simulink model "pid_10"  (R2022a)
settings: Solver=FixedStepAuto  StartTime=0.0  StopTime=12.0  FixedStep=0.1  RelTol=1e-3  EnableMultiTasking=on
libraries: mbedblockslib x27, simulink x3, hdlsllib x2, slctrlblks x1, slpidlib x1
(part 1 of 2)
settings Model: PacingRate=0.750000  ExtModeTrigDuration=10  Creator=MATLAB  LastModifiedBy=FUGAZI
settings SolverCC: AutoInsertRateTranBlk=on
settings OptimizationCC: EnhancedBackFolding=on  PassReuseOutputArgsAs=Individual arguments  ZeroExternalMemoryAtStartup=off  ZeroInternalMemoryAtStartup=off  MaxStackSize=64  OptimizeBlockOrder=speed  DifferentSizesBufferReuse=on  OptimizationCustomize=off  EfficientTunableParamExpr=on
settings DebuggingCC: ParameterTunabilityLossMsg=error
settings HardwareCC: ProdBitPerPointer=32  ProdBitPerSizeT=32  ProdBitPerPtrDiffT=32  ProdLargestAtomicInteger=Long  ProdLargestAtomicFloat=Double  ProdWordSize=32  ProdLongLongMode=on  ProdHWDeviceType=ARM Compatible->ARM Cortex
settings SFSimCC: MATLABDynamicMemAlloc=off
settings RTWCC: SystemTargetFile=ert.tlc  HardwareBoard=STM32 Nucleo L476RG  TemplateMakefile=ert_default_tmf  Toolchain=GNU Tools for ARM Embedded Processors
settings CodeAppCC: ForceParamTrailComments=on  IgnoreCustomStorageClasses=off  OperatorAnnotations=on  SimulinkDataObjDesc=on  SFDataObjDesc=on  InsertBlockDesc=on
settings ERTTargetCC: SupportContinuousTime=on  ExtModeTransport=3  ExtModeStaticAlloc=on  ExtModeStaticAllocSize=2000  ExtModeMexFile=ext_xcp  ExtModeIntrfLevel=Level2 - Open

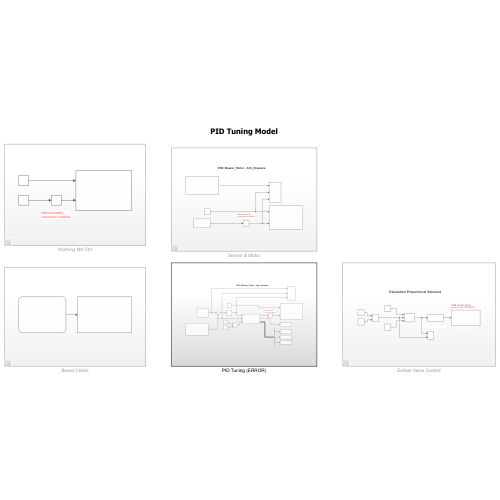
[thumbnail: Simulink's stored preview of the top-level diagram]
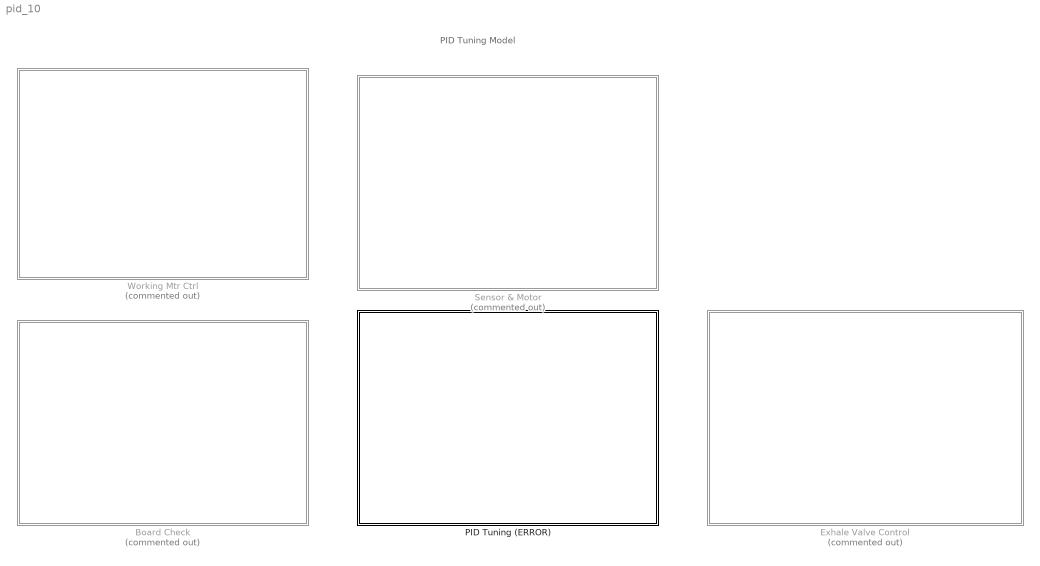
== system pid_10 ==
  note: PID Tuning Model
  Board Check : Subsystem  Commented=on
  Exhale Valve Control : Subsystem  Commented=on
  PID Tuning (ERROR) : Subsystem
  Sensor & Motor : Subsystem  Commented=on
  Working Mtr Ctrl : Subsystem  Commented=on

== system pid_10/Board Check ==
  Start-Up : Stateflow chart  TreatAsAtomicUnit=on
  SubSystem Relays : Subsystem
  wires:
  Start-Up/1(LED) -> SubSystem Relays/1(LED)

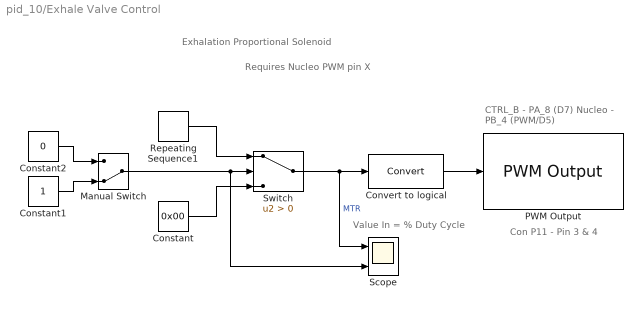
== system pid_10/Exhale Valve Control ==
  note: Exhalation Proportional Solenoid
  note: Value In = % Duty Cycle
  note: Con P11 - Pin 3 & 4
  note: Requires Nucleo PWM pin X
  note: CTRL_B - PA_8 (D7)
      | Nucleo - PB_4 (PWM/D5)
  Constant : Constant  Value=0x00
  Constant1 : Constant
  Constant2 : Constant  Value=0
  Convert to logical : DataTypeConversion  SaturateOnIntegerOverflow=off  RndMeth=Floor
  Manual Switch : ManualSwitch  CurrentSetting=0
  PWM Output : mbedblockslib/PWM Output  Pin=PB_4  EnableInputFrequency=off  InitialFrequency=500  InitialDutyCycle=85  NotificationType=None
      settings: SourceProductBaseCode=MICROBIT,NUCLEO,STMICRODIS
  Repeating Sequence1 : simulink/Sources/Repeating Sequence  rep_seq_t=[0 1.3 1.4 2.5 2.6]  rep_seq_y=[15 15 71 71 15]
  Scope : Scope  NumInputPorts=2
  Switch : Switch  Criteria=u2 > Threshold  SaturateOnIntegerOverflow=off  InputSameDT=off
  wires:
  Manual Switch/1 -> Scope/2, Switch/2
  Convert to logical/1 -> PWM Output/1
  Switch/1 -> Scope/1, Convert to logical/1  "MTR"
  Repeating Sequence1/1 -> Switch/1
  Constant/1 -> Switch/3
  Constant1/1 -> Manual Switch/2
  Constant2/1 -> Manual Switch/1

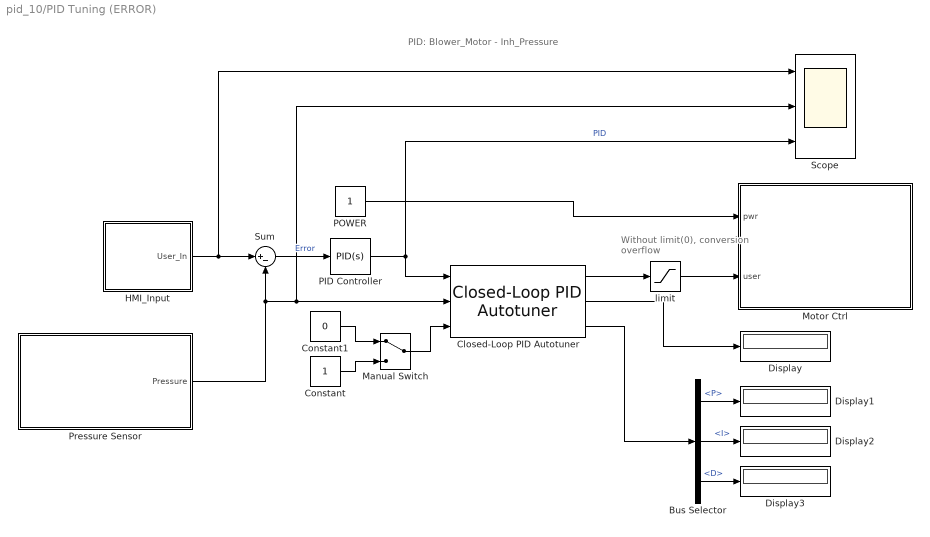
== system pid_10/PID Tuning (ERROR) ==
  note: Without limit(0),
      | conversion overflow
  note: PID: Blower_Motor - Inh_Pressure
  Bus Selector : BusSelector  OutputSignals=P,I,D
  Closed-Loop PID Autotuner : slctrlblks/Closed-Loop PID Autotuner  PIDType=PI  PIDForm=Parallel  TimeDomain=discrete-time  DiscreteTs=0.1  TuningTs=0.2  UseTuningTs=off  IntegratorFormula=Forward Euler  FilterFormula=Forward Euler  ContinuousTs=0.02  Bandwidth=1  UseExternalWC=off  TargetPM=60  UseExternalPM=off  UseExternalAchievedPM=off  ExperimentMode=Superposition  PlantType=Stable  PlantSign=Positive  AmpSine=1  UseExternalAmpSine=off  UseExternalFRD=off  UseExternalU0=off  UseCompanion=off  NotDeployTuningModule=off  UsePLCCoder=off  OutputMode=control action + perturbation  BlockDataType=double  UseConnectedPID=on  blockpath=[]  tunedP=0  tunedI=0  tunedD=0  tunedN=100  tunedPM=0  EstimationWindowSize=3  UseExternalTuningParams=off  OutputChoice=VariantCandD  SingleMultiRateVariant=SingleSamplingRate  ExperimentModeVariant=VariantSuperimposed  NumEstimationPeriods=4  NumSettlingPeriods=2
      settings: SourceProductBaseCode=SD
  Constant : Constant
  Constant1 : Constant  Value=0
  Display{,1..3} (4 alike) : Display
  HMI_Input : Subsystem
  Manual Switch : ManualSwitch
  Motor Ctrl : Subsystem
  PID Controller : slpidlib/PID Controller  Controller=PID  Form=Parallel  TimeDomain=Continuous-time  UseExternalTs=off  SampleTime=-1  IntegratorMethod=Forward Euler  FilterMethod=Forward Euler  ControllerParametersSource=internal  P=2  I=2  UseKiTs=off  D=1.5  N=280  UseFilter=on  TunerSelectOption=Transfer Function Based (PID Tuner App)  InitialConditionSource=internal  InitialConditionForIntegrator=0  InitialConditionForFilter=0  DifferentiatorICPrevScaledInput=0  ExternalReset=none  TrackingMode=off  Kt=1  LimitOutput=off  SatLimitsSource=internal  UpperSaturationLimit=inf  LowerSaturationLimit=-inf  LinearizeAsGain=on  AntiWindupMode=none  Kb=1  POutMin=[]  POutMax=[]  IOutMin=[]  IOutMax=[]  DOutMin=[]  DOutMax=[]  NOutMin=[]  NOutMax=[]  SumOutMin=[]  SumOutMax=[]  SaturationOutMin=[]  SaturationOutMax=[]  PParamMin=[]  PParamMax=[]  IParamMin=[]  IParamMax=[]  DParamMin=[]  DParamMax=[]  NParamMin=[]  NParamMax=[]  KbParamMin=[]  KbParamMax=[]  KtParamMin=[]  KtParamMax=[]  KbOutMin=[]  KbOutMax=[]  KtOutMin=[]  KtOutMax=[]  IntegratorOutMin=[]  IntegratorOutMax=[]  FilterOutMin=[]  FilterOutMax=[]  SumI1OutMin=[]  SumI1OutMax=[]  SumI2OutMin=[]  SumI2OutMax=[]  SumI3OutMin=[]  SumI3OutMax=[]  SumI4OutMin=[]  SumI4OutMax=[]  SumDOutMin=[]  SumDOutMax=[]  DifferentiatorOutMin=[]  DifferentiatorOutMax=[]  FilterDiffOutCoefMin=[]  FilterDiffOutCoefMax=[]  ReciprocalOutMin=[]  ReciprocalOutMax=[]  SumDenOutMin=[]  SumDenOutMax=[]  SumNumOutMin=[]  SumNumOutMax=[]  DivideOutMin=[]  DivideOutMax=[]  UdiffTsProdOutMin=[]  UdiffTsProdOutMax=[]  NTsProdOutMin=[]  NTsProdOutMax=[]  UintegralTsProdOutMin=[]  UintegralTsProdOutMax=[]  UngainTsProdOutMin=[]  UngainTsProdOutMax=[]  IntegratorContinuousStateAttributes=''  IntegratorStateMustResolveToSignalObject=off  IntegratorRTWStateStorageClass=Auto  FilterContinuousStateAttributes=''  FilterStateMustResolveToSignalObject=off  FilterRTWStateStorageClass=Auto  ParallelPVariant=InternalParameters  IdealPVariant=Disabled  IVariant=InternalParameters  DVariant=InternalParameters  IntegratorVariant=Continuous  SatVariant=Disabled  AWVariant=Passthrough  PCopyVariant=Disabled  TRVariant=Disabled  FdbkBlocksVariant=Forward  IdealPFdbkVariant=Disabled  SatFdbkVariant=Disabled  DerivativeFilterVariant=ContFilter  NVariant=InternalParameters  NCopyVariant=Disabled  FilterICVariant=InternalICsFilter  IntegratorICVariant=InternalICs  ExternalResetVariant=Disabled  TRSumVariant=Passthrough  SumFdbkVariant=Disabled  SumVariant=Sum_PID  TsampFilterVariant=InternalTs  TsampNgainVariant=Passthrough  TsampIntegralVariant=Passthrough  ExternalSaturationOutDataTypeStr=Inherit: Same as second input  aMode=0
  POWER : Constant
  Pressure Sensor : Subsystem
  Scope : Scope  NumInputPorts=3
  Sum : Sum  Inputs=|+-
  limit : Saturate  UpperLimit=254  LowerLimit=0
  wires:
  POWER/1 -> Motor Ctrl/1(pwr)
  Bus Selector/3 -> Display3/1  "<D>"
  Pressure Sensor/1(Pressure) -> Sum/2, Scope/2, Closed-Loop PID Autotuner/2
  Closed-Loop PID Autotuner/2 -> Display/1
  Closed-Loop PID Autotuner/1 -> limit/1
  Constant1/1 -> Manual Switch/1
  Bus Selector/2 -> Display2/1  "<I>"
  Bus Selector/1 -> Display1/1  "<P>"
  HMI_Input/1(User_In) -> Scope/1, Sum/1
  Closed-Loop PID Autotuner/3 -> Bus Selector/1
  Manual Switch/1 -> Closed-Loop PID Autotuner/3
  PID Controller/1 -> Closed-Loop PID Autotuner/1, Scope/3  "PID"
  Constant/1 -> Manual Switch/2
  Sum/1 -> PID Controller/1  "Error"
  limit/1 -> Motor Ctrl/2(user)

== system pid_10/Sensor & Motor ==
  note: PID: Blower_Motor - Inh_Pressure
  note: Without limit(0),
      | conversion overflow
  HMI_Input : Subsystem
  Motor Ctrl : Subsystem
  POWER : Constant
  Pressure Sensor : Subsystem
  Scope : Scope  NumInputPorts=3
  limit : Saturate  UpperLimit=254  LowerLimit=0
  wires:
  limit/1 -> Scope/3, Motor Ctrl/2(user)
  POWER/1 -> Scope/2, Motor Ctrl/1(pwr)
  HMI_Input/1(User_In) -> limit/1
  Pressure Sensor/1(Pressure) -> Scope/1

== system pid_10/Working Mtr Ctrl ==
  note: Without limit(0),
      | conversion overflow
  Constant : Constant
  Constant1 : Constant  Value=120
  Motor Ctrl : Subsystem
  limit : Saturate  UpperLimit=254  LowerLimit=0
  wires:
  limit/1 -> Motor Ctrl/2(user)
  Constant1/1 -> limit/1
  Constant/1 -> Motor Ctrl/1(pwr)

== system pid_10/Board Check/SubSystem Relays ==
  note: Logic Switching Sub-Systems
  note: Simulation Port
  note: Status LED PB_0
      | Nucleo PA_5
  LED : Inport
  Data Type Conversion1 : DataTypeConversion  SaturateOnIntegerOverflow=off  RndMeth=Floor
  Digital Write2 : mbedblockslib/Digital Write  Pin=PA_5  Direction=output
      settings: SourceProductBaseCode=MICROBIT,NUCLEO,STMICRODIS
  Scope : Scope
  wires:
  LED/1 -> Data Type Conversion1/1
  Data Type Conversion1/1 -> Digital Write2/1, Scope/1

== system pid_10/PID Tuning (ERROR)/HMI_Input ==
  Constant : Constant  Value=8
  Continuous Input : DiscretePulseGenerator  Commented=on  PulseType=Time based  Amplitude=61  Period=10  PulseWidth=50
  Step Input : Step  Before=6  After=21  SampleTime=5
  Varying Inputs : simulink/Sources/Repeating Sequence Stair  Commented=on  OutValues=[1638 8191 16383 8191 1638].'  tsamp=2  OutMin=[]  OutMax=[]  OutDataTypeStr=double  OutputDataTypeScalingMode=double  OutDataType=fixdt(0,8)  ConRadixGroup=Best Precision: Vector-wise  OutScaling=2^-12
  User_In : Outport
  wires:
  Constant/1 -> User_In/1

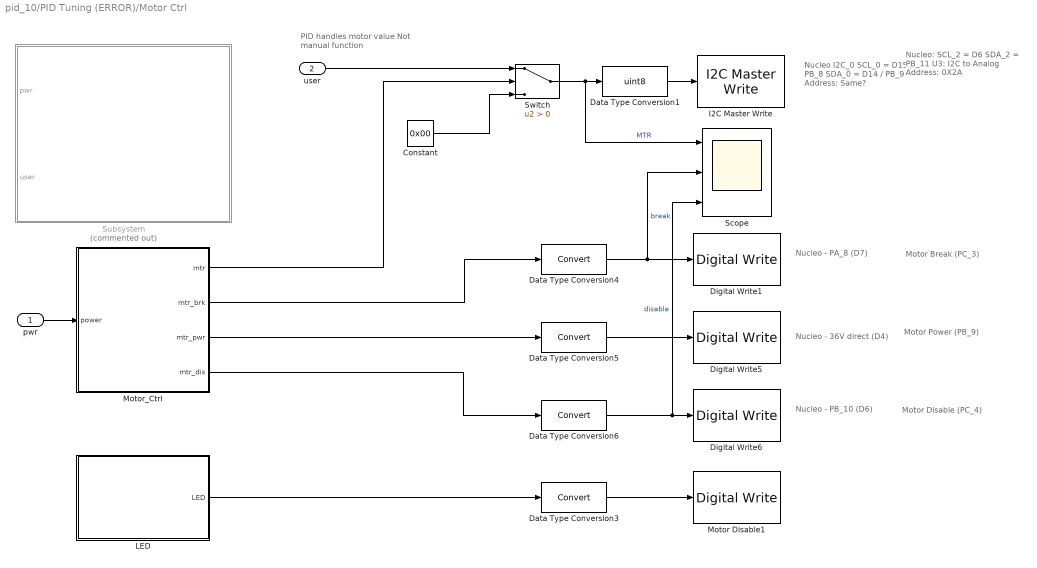
== system pid_10/PID Tuning (ERROR)/Motor Ctrl ==
  note: Nucleo I2C_0
      | SCL_0 = D15 / PB_8
      | SDA_0 = D14 / PB_9
      | Address: Same?
  note: PID handles motor value
      | Not manual function
  note: Motor Power
      | (PB_9)
  note: Motor Break
      | (PC_3)
  note: Nucleo:
      | SCL_2 = D6
      | SDA_2 = PB_11
      | U3: I2C to Analog
      | Address: 0X2A
  note: Nucleo - 36V direct
      | (D4)
  note: Motor Disable
      | (PC_4)
  note: Nucleo - PA_8
      | (D7)
  note: Nucleo - PB_10
      | (D6)
  pwr : Inport
  user : Inport  Port=2
  Constant : Constant  Value=0x00
  Data Type Conversion1 : DataTypeConversion  OutDataTypeStr=uint8  SaturateOnIntegerOverflow=off  RndMeth=Floor
  Data Type Conversion{3..6} (4 alike) : DataTypeConversion  SaturateOnIntegerOverflow=off  RndMeth=Floor
  Digital Write1 : mbedblockslib/Digital Write  Pin=PA_8  Direction=output
      settings: SourceProductBaseCode=MICROBIT,NUCLEO,STMICRODIS
  Digital Write5 : mbedblockslib/Digital Write  Pin=PB_5  Direction=output
      settings: SourceProductBaseCode=MICROBIT,NUCLEO,STMICRODIS
  Digital Write6 : mbedblockslib/Digital Write  Pin=PB_10  Direction=output
      settings: SourceProductBaseCode=MICROBIT,NUCLEO,STMICRODIS
  I2C Master Write : mbedblockslib/I2C Master Write  I2CModule=0  Mode=Master  SlaveAddress=uint8(hex2dec('2A'))  SlaveByteOrder=BigEndian  Direction=Transmitter  RegisterAddressMode=on  RegisterAddress=uint8(hex2dec('10'))  SlaveDataType=uint8  DataLength=2  NoAck=off  RepeatedStart=off  OutputStatus=off
      settings: SourceProductBaseCode=MICROBIT,NUCLEO,STMICRODIS
  LED : Stateflow chart  TreatAsAtomicUnit=on
  Motor Disable1 : mbedblockslib/Digital Write  Pin=PA_5  Direction=output
      settings: SourceProductBaseCode=MICROBIT,NUCLEO,STMICRODIS
  Motor_Ctrl : Stateflow chart  TreatAsAtomicUnit=on
  Scope : Scope  NumInputPorts=3
  Subsystem : Subsystem  Commented=on
  Switch : Switch  Criteria=u2 > Threshold  SaturateOnIntegerOverflow=off  InputSameDT=off
  wires:
  Motor_Ctrl/3(mtr_pwr) -> Data Type Conversion5/1
  Constant/1 -> Switch/3
  Data Type Conversion3/1 -> Motor Disable1/1
  LED/1(LED) -> Data Type Conversion3/1
  Switch/1 -> Scope/1, Data Type Conversion1/1  "MTR"
  user/1 -> Switch/1
  Data Type Conversion5/1 -> Digital Write5/1
  Data Type Conversion4/1 -> Scope/2, Digital Write1/1  "break"
  pwr/1 -> Motor_Ctrl/1(power)
  Motor_Ctrl/1(mtr) -> Switch/2
  Data Type Conversion6/1 -> Scope/3, Digital Write6/1  "disable"
  Motor_Ctrl/4(mtr_dis) -> Data Type Conversion6/1
  Data Type Conversion1/1 -> I2C Master Write/1
  Motor_Ctrl/2(mtr_brk) -> Data Type Conversion4/1

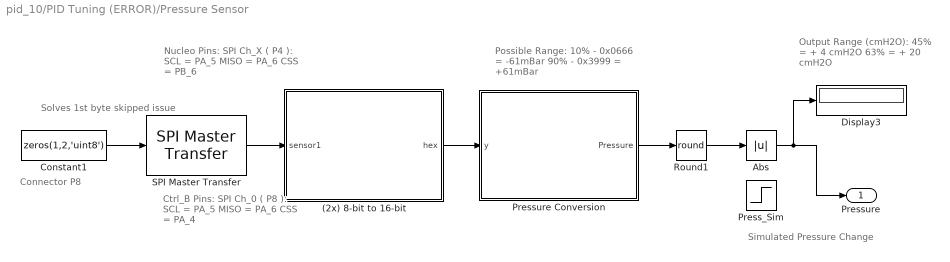
== system pid_10/PID Tuning (ERROR)/Pressure Sensor ==
  note: Ctrl_B Pins:
      | SPI Ch_0 ( P8 ):
      | SCL = PA_5
      | MISO = PA_6
      | CSS = PA_4
  note: Possible Range:
      | 10% - 0x0666 = -61mBar
      | 90% - 0x3999 = +61mBar
  note: Connector P8
  note: Solves 1st byte
      | skipped issue
  note: Output Range (cmH2O):
      | 45% = + 4 cmH2O
      | 63% = + 20 cmH2O
  note: Simulated Pressure Change
  note: Nucleo Pins:
      | SPI Ch_X ( P4 ):
      | SCL = PA_5
      | MISO = PA_6
      | CSS = PB_6
  (2x) 8-bit to 16-bit : Subsystem
  Abs : Abs  SaturateOnIntegerOverflow=off
  Constant1 : Constant  Value=zeros(1,2,'uint8')  OutDataTypeStr=uint8  SampleTime=0.1
  Display3 : Display
      settings: Format=hex (Stored Integer)
  Press_Sim : Step  Before=6  After=12  SampleTime=5
  Pressure Conversion : Subsystem
  Round1 : Rounding  Operator=round
  SPI Master Transfer : mbedblockslib/SPI Master Transfer  SPIModule=0  Mode=Master  BusSpeed=uint32( 1000000 )  Pin=PB_6  FirstBitToTransfer=Most significant bit (MSB)  ClockMode=0  BlockFunction=Transfer  RegisterAddress=0  OutputDataType=int8  OutputDataLength=1  UseCustomSSPin=Explicit GPIO calls  ActiveLowSSPin=Active low
      settings: SourceProductBaseCode=MICROBIT,NUCLEO,STMICRODIS
  Pressure : Outport
  wires:
  Pressure Conversion/1(Pressure) -> Round1/1
  Constant1/1 -> SPI Master Transfer/1
  Round1/1 -> Abs/1
  Abs/1 -> Pressure/1, Display3/1
  SPI Master Transfer/1 -> (2x) 8-bit to 16-bit/1(sensor1)
  (2x) 8-bit to 16-bit/1(hex) -> Pressure Conversion/1(y)

== system pid_10/Sensor & Motor/HMI_Input ==
  Constant : Constant  Value=120
  Continuous Input : DiscretePulseGenerator  Commented=on  PulseType=Time based  Amplitude=61  Period=10  PulseWidth=50
  Step Input : Step  Before=6  After=21  SampleTime=5
  Varying Inputs : simulink/Sources/Repeating Sequence Stair  Commented=on  OutValues=[1638 8191 16383 8191 1638].'  tsamp=2  OutMin=[]  OutMax=[]  OutDataTypeStr=double  OutputDataTypeScalingMode=double  OutDataType=fixdt(0,8)  ConRadixGroup=Best Precision: Vector-wise  OutScaling=2^-12
  User_In : Outport
  wires:
  Constant/1 -> User_In/1

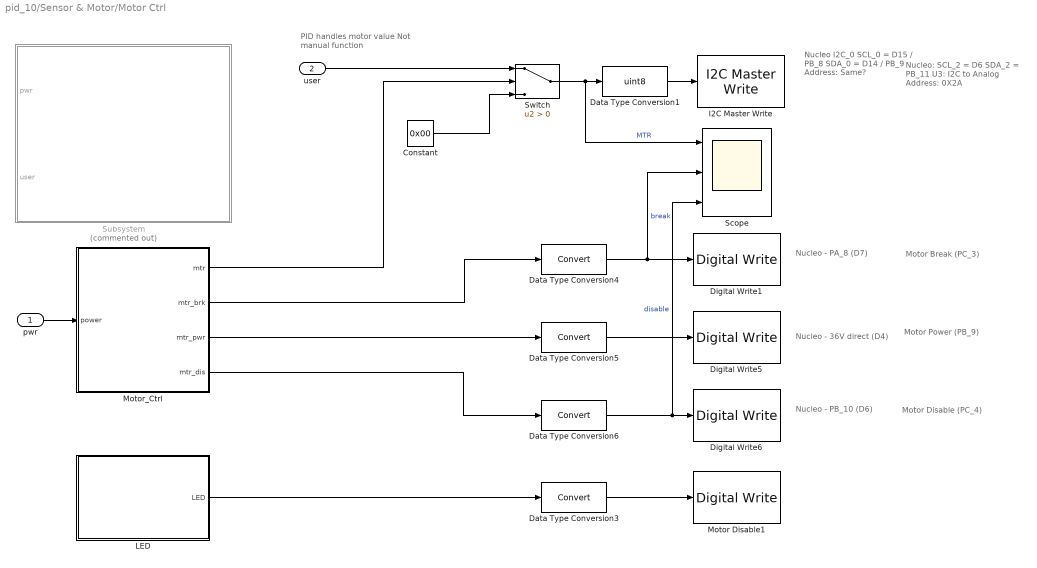
== system pid_10/Sensor & Motor/Motor Ctrl ==
  note: Nucleo - PB_10
      | (D6)
  note: Nucleo - PA_8
      | (D7)
  note: Motor Disable
      | (PC_4)
  note: Nucleo - 36V direct
      | (D4)
  note: Nucleo:
      | SCL_2 = D6
      | SDA_2 = PB_11
      | U3: I2C to Analog
      | Address: 0X2A
  note: Motor Break
      | (PC_3)
  note: Motor Power
      | (PB_9)
  note: PID handles motor value
      | Not manual function
  note: Nucleo I2C_0
      | SCL_0 = D15 / PB_8
      | SDA_0 = D14 / PB_9
      | Address: Same?
  pwr : Inport
  user : Inport  Port=2
  Constant : Constant  Value=0x00
  Data Type Conversion1 : DataTypeConversion  OutDataTypeStr=uint8  SaturateOnIntegerOverflow=off  RndMeth=Floor
  Data Type Conversion{3..6} (4 alike) : DataTypeConversion  SaturateOnIntegerOverflow=off  RndMeth=Floor
  Digital Write1 : mbedblockslib/Digital Write  Pin=PA_8  Direction=output
      settings: SourceProductBaseCode=MICROBIT,NUCLEO,STMICRODIS
  Digital Write5 : mbedblockslib/Digital Write  Pin=PB_5  Direction=output
      settings: SourceProductBaseCode=MICROBIT,NUCLEO,STMICRODIS
  Digital Write6 : mbedblockslib/Digital Write  Pin=PB_10  Direction=output
      settings: SourceProductBaseCode=MICROBIT,NUCLEO,STMICRODIS
  I2C Master Write : mbedblockslib/I2C Master Write  I2CModule=0  Mode=Master  SlaveAddress=uint8(hex2dec('2A'))  SlaveByteOrder=BigEndian  Direction=Transmitter  RegisterAddressMode=on  RegisterAddress=uint8(hex2dec('10'))  SlaveDataType=uint8  DataLength=2  NoAck=off  RepeatedStart=off  OutputStatus=off
      settings: SourceProductBaseCode=MICROBIT,NUCLEO,STMICRODIS
  LED : Stateflow chart  TreatAsAtomicUnit=on
  Motor Disable1 : mbedblockslib/Digital Write  Pin=PA_5  Direction=output
      settings: SourceProductBaseCode=MICROBIT,NUCLEO,STMICRODIS
  Motor_Ctrl : Stateflow chart  TreatAsAtomicUnit=on
  Scope : Scope  NumInputPorts=3
  Subsystem : Subsystem  Commented=on
  Switch : Switch  Criteria=u2 > Threshold  SaturateOnIntegerOverflow=off  InputSameDT=off
  wires:
  Motor_Ctrl/2(mtr_brk) -> Data Type Conversion4/1
  Data Type Conversion1/1 -> I2C Master Write/1
  Motor_Ctrl/4(mtr_dis) -> Data Type Conversion6/1
  Data Type Conversion6/1 -> Digital Write6/1, Scope/3  "disable"
  Motor_Ctrl/1(mtr) -> Switch/2
  pwr/1 -> Motor_Ctrl/1(power)
  Data Type Conversion4/1 -> Digital Write1/1, Scope/2  "break"
  Data Type Conversion5/1 -> Digital Write5/1
  user/1 -> Switch/1
  Switch/1 -> Data Type Conversion1/1, Scope/1  "MTR"
  LED/1(LED) -> Data Type Conversion3/1
  Data Type Conversion3/1 -> Motor Disable1/1
  Constant/1 -> Switch/3
  Motor_Ctrl/3(mtr_pwr) -> Data Type Conversion5/1

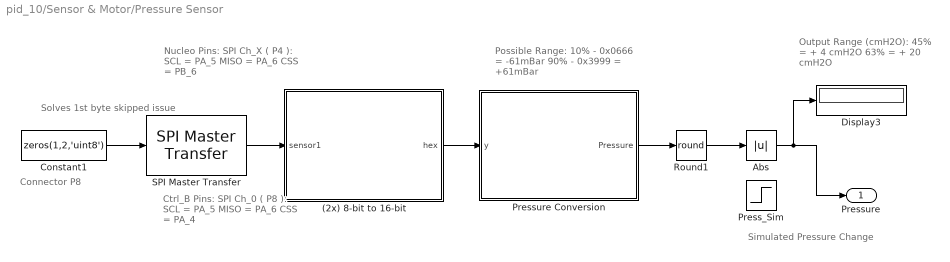
== system pid_10/Sensor & Motor/Pressure Sensor ==
  note: Nucleo Pins:
      | SPI Ch_X ( P4 ):
      | SCL = PA_5
      | MISO = PA_6
      | CSS = PB_6
  note: Simulated Pressure Change
  note: Output Range (cmH2O):
      | 45% = + 4 cmH2O
      | 63% = + 20 cmH2O
  note: Solves 1st byte
      | skipped issue
  note: Connector P8
  note: Possible Range:
      | 10% - 0x0666 = -61mBar
      | 90% - 0x3999 = +61mBar
  note: Ctrl_B Pins:
      | SPI Ch_0 ( P8 ):
      | SCL = PA_5
      | MISO = PA_6
      | CSS = PA_4
  (2x) 8-bit to 16-bit : Subsystem
  Abs : Abs  SaturateOnIntegerOverflow=off
  Constant1 : Constant  Value=zeros(1,2,'uint8')  OutDataTypeStr=uint8  SampleTime=0.1
  Display3 : Display
      settings: Format=hex (Stored Integer)
  Press_Sim : Step  Before=6  After=12  SampleTime=5
  Pressure Conversion : Subsystem
  Round1 : Rounding  Operator=round
  SPI Master Transfer : mbedblockslib/SPI Master Transfer  SPIModule=0  Mode=Master  BusSpeed=uint32( 1000000 )  Pin=PB_6  FirstBitToTransfer=Most significant bit (MSB)  ClockMode=0  BlockFunction=Transfer  RegisterAddress=0  OutputDataType=int8  OutputDataLength=1  UseCustomSSPin=Explicit GPIO calls  ActiveLowSSPin=Active low
      settings: SourceProductBaseCode=MICROBIT,NUCLEO,STMICRODIS
  Pressure : Outport
  wires:
  (2x) 8-bit to 16-bit/1(hex) -> Pressure Conversion/1(y)
  SPI Master Transfer/1 -> (2x) 8-bit to 16-bit/1(sensor1)
  Abs/1 -> Display3/1, Pressure/1
  Round1/1 -> Abs/1
  Constant1/1 -> SPI Master Transfer/1
  Pressure Conversion/1(Pressure) -> Round1/1

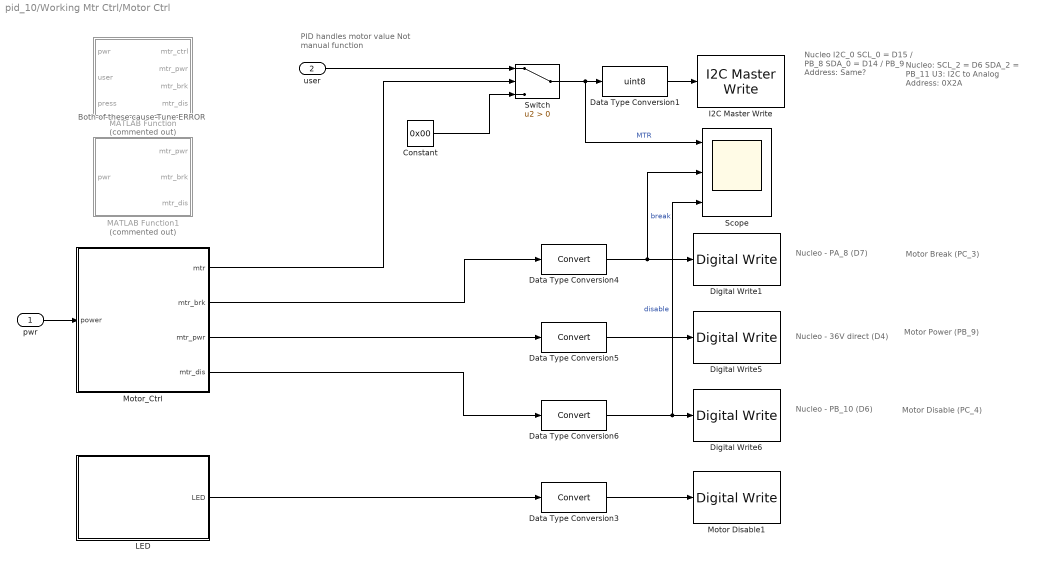
== system pid_10/Working Mtr Ctrl/Motor Ctrl ==
  note: Both of these cause Tune ERROR
  note: PID handles motor value
      | Not manual function
  note: Nucleo:
      | SCL_2 = D6
      | SDA_2 = PB_11
      | U3: I2C to Analog
      | Address: 0X2A
  note: Motor Break
      | (PC_3)
  note: Nucleo - 36V direct
      | (D4)
  note: Nucleo - PA_8
      | (D7)
  note: Motor Power
      | (PB_9)
  note: Nucleo - PB_10
      | (D6)
  note: Motor Disable
      | (PC_4)
  note: Nucleo I2C_0
      | SCL_0 = D15 / PB_8
      | SDA_0 = D14 / PB_9
      | Address: Same?
  pwr : Inport
  user : Inport  Port=2
  Constant : Constant  Value=0x00
  Data Type Conversion1 : DataTypeConversion  OutDataTypeStr=uint8  SaturateOnIntegerOverflow=off  RndMeth=Floor
  Data Type Conversion{3..6} (4 alike) : DataTypeConversion  SaturateOnIntegerOverflow=off  RndMeth=Floor
  Digital Write1 : mbedblockslib/Digital Write  Pin=PA_8  Direction=output
      settings: SourceProductBaseCode=MICROBIT,NUCLEO,STMICRODIS
  Digital Write5 : mbedblockslib/Digital Write  Pin=PB_5  Direction=output
      settings: SourceProductBaseCode=MICROBIT,NUCLEO,STMICRODIS
  Digital Write6 : mbedblockslib/Digital Write  Pin=PB_10  Direction=output
      settings: SourceProductBaseCode=MICROBIT,NUCLEO,STMICRODIS
  I2C Master Write : mbedblockslib/I2C Master Write  I2CModule=0  Mode=Master  SlaveAddress=uint8(hex2dec('2A'))  SlaveByteOrder=BigEndian  Direction=Transmitter  RegisterAddressMode=on  RegisterAddress=uint8(hex2dec('10'))  SlaveDataType=uint8  DataLength=2  NoAck=off  RepeatedStart=off  OutputStatus=off
      settings: SourceProductBaseCode=MICROBIT,NUCLEO,STMICRODIS
  LED : Stateflow chart  TreatAsAtomicUnit=on
  MATLAB Function : MATLAB Function  Commented=on  TreatAsAtomicUnit=on
  MATLAB Function1 : MATLAB Function  Commented=on  TreatAsAtomicUnit=on
  Motor Disable1 : mbedblockslib/Digital Write  Pin=PA_5  Direction=output
      settings: SourceProductBaseCode=MICROBIT,NUCLEO,STMICRODIS
  Motor_Ctrl : Stateflow chart  TreatAsAtomicUnit=on
  Scope : Scope  NumInputPorts=3
  Switch : Switch  Criteria=u2 > Threshold  SaturateOnIntegerOverflow=off  InputSameDT=off
  wires:
  Data Type Conversion1/1 -> I2C Master Write/1
  Motor_Ctrl/2(mtr_brk) -> Data Type Conversion4/1
  LED/1(LED) -> Data Type Conversion3/1
  Motor_Ctrl/3(mtr_pwr) -> Data Type Conversion5/1
  Motor_Ctrl/4(mtr_dis) -> Data Type Conversion6/1
  Data Type Conversion5/1 -> Digital Write5/1
  Data Type Conversion4/1 -> Scope/2, Digital Write1/1  "break"
  Data Type Conversion6/1 -> Scope/3, Digital Write6/1  "disable"
  Data Type Conversion3/1 -> Motor Disable1/1
  pwr/1 -> Motor_Ctrl/1(power)
  Constant/1 -> Switch/3
  Switch/1 -> Scope/1, Data Type Conversion1/1  "MTR"
  Motor_Ctrl/1(mtr) -> Switch/2
  user/1 -> Switch/1

== system pid_10/PID Tuning (ERROR)/Motor Ctrl/Subsystem ==
  note: PID handles motor value
      | Not manual function
  note: SCL_2 = D6
      | SDA_2 = PB_11
      | U3: I2C to Analog
      | Address: 0X2A
  note: Motor Break
  note: Motor Disable
  note: Motor Power
  pwr : Inport
  user : Inport  Port=2
  Data Type Conversion1 : DataTypeConversion  OutDataTypeStr=uint8  SaturateOnIntegerOverflow=off  RndMeth=Floor
  MATLAB Function : MATLAB Function  Commented=on  TreatAsAtomicUnit=on
  MATLAB Function1 : MATLAB Function  TreatAsAtomicUnit=on
  Motor Break : mbedblockslib/Digital Write  Pin=PB_0  Direction=output
      settings: SourceProductBaseCode=MICROBIT,NUCLEO,STMICRODIS
  Motor Disable : mbedblockslib/Digital Write  Pin=PB_0  Direction=output
      settings: SourceProductBaseCode=MICROBIT,NUCLEO,STMICRODIS
  Motor Power : mbedblockslib/Digital Write  Pin=PB_0  Direction=output
      settings: SourceProductBaseCode=MICROBIT,NUCLEO,STMICRODIS
  Motor Speed Control : mbedblockslib/I2C Master Write  I2CModule=2  Mode=Master  SlaveAddress=uint8(hex2dec('2A'))  SlaveByteOrder=BigEndian  Direction=Transmitter  RegisterAddressMode=on  RegisterAddress=uint8(hex2dec('10'))  SlaveDataType=uint8  DataLength=2  NoAck=off  RepeatedStart=off  OutputStatus=off
      settings: SourceProductBaseCode=MICROBIT,NUCLEO,STMICRODIS
  wires:
  user/1 -> Data Type Conversion1/1
  MATLAB Function1/1(mtr_pwr) -> Motor Power/1
  MATLAB Function1/2(mtr_brk) -> Motor Break/1
  pwr/1 -> MATLAB Function1/1(pwr)
  Data Type Conversion1/1 -> Motor Speed Control/1
  MATLAB Function1/3(mtr_dis) -> Motor Disable/1

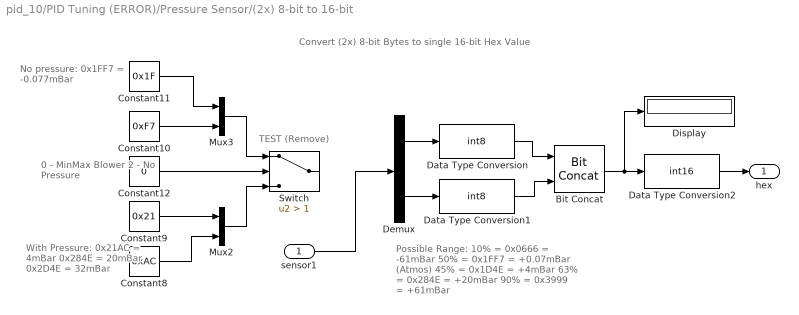
== system pid_10/PID Tuning (ERROR)/Pressure Sensor/(2x) 8-bit to 16-bit ==
  note: Convert (2x) 8-bit Bytes to single 16-bit Hex Value
  note: 0 - MinMax Blower
      | 2 - No Pressure
  note: No pressure:
      | 0x1FF7 = -0.077mBar
  note: Possible Range:
      | 10% = 0x0666 = -61mBar
      | 50% = 0x1FF7 = +0.07mBar (Atmos)
      | 45% = 0x1D4E = +4mBar
      | 63% = 0x284E = +20mBar
      | 90% = 0x3999 = +61mBar
  note: With Pressure:
      | 0x21AC = 4mBar
      | 0x284E = 20mBar
      | 0x2D4E = 32mBar
  note: TEST (Remove)
  sensor1 : Inport
  Bit Concat : hdlsllib/Logic and Bit Operations/Bit Concat  numInputs=2
  Constant10 : Constant  Value=0xF7
  Constant11 : Constant  Value=0x1F
  Constant12 : Constant  Value=0
  Constant8 : Constant  Value=0xAC
  Constant9 : Constant  Value=0x21
  Data Type Conversion : DataTypeConversion  OutDataTypeStr=int8  SaturateOnIntegerOverflow=off  RndMeth=Floor
  Data Type Conversion1 : DataTypeConversion  OutDataTypeStr=int8  SaturateOnIntegerOverflow=off  RndMeth=Floor
  Data Type Conversion2 : DataTypeConversion  OutDataTypeStr=int16  SaturateOnIntegerOverflow=off  RndMeth=Floor
  Demux : Demux  Outputs=2
  Display : Display
      settings: Format=hex (Stored Integer)
  Mux2 : Mux  Inputs=2
  Mux3 : Mux  Inputs=2
  Switch : Switch  Criteria=u2 > Threshold  Threshold=1  SaturateOnIntegerOverflow=off  InputSameDT=off
  hex : Outport
  wires:
  Data Type Conversion/1 -> Bit Concat/1
  Data Type Conversion1/1 -> Bit Concat/2
  Demux/1 -> Data Type Conversion/1
  Demux/2 -> Data Type Conversion1/1
  Bit Concat/1 -> Display/1, Data Type Conversion2/1
  Constant9/1 -> Mux2/1
  Constant8/1 -> Mux2/2
  Constant10/1 -> Mux3/2
  Constant11/1 -> Mux3/1
  Constant12/1 -> Switch/2
  Mux3/1 -> Switch/1
  Mux2/1 -> Switch/3
  Data Type Conversion2/1 -> hex/1
  sensor1/1 -> Demux/1

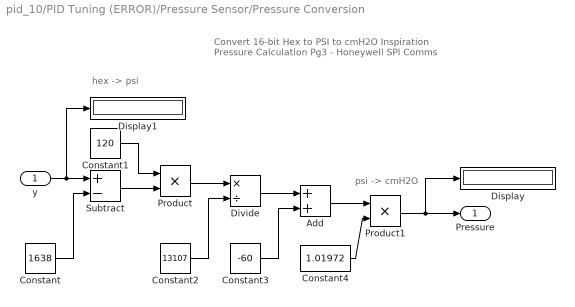
== system pid_10/PID Tuning (ERROR)/Pressure Sensor/Pressure Conversion ==
  note: psi -> cmH2O
  note: Convert 16-bit Hex to PSI to cmH2O
      | Inspiration Pressure Calculation
      | Pg3 - Honeywell SPI Comms
  note: hex -> psi
  y : Inport
  Add : Sum
  Constant : Constant  Value=1638
  Constant1 : Constant  Value=120
  Constant2 : Constant  Value=13107
  Constant3 : Constant  Value=-60
  Constant4 : Constant  Value=1.01972
  Display : Display
  Display1 : Display
      settings: Format=hex (Stored Integer)
  Divide : Product  Inputs=*/
  Product : Product
  Product1 : Product
  Subtract : Sum  Inputs=+-
  Pressure : Outport
  wires:
  Constant/1 -> Subtract/2
  Subtract/1 -> Product/2
  Constant1/1 -> Product/1
  Product/1 -> Divide/1
  Constant2/1 -> Divide/2
  Constant3/1 -> Add/2
  Divide/1 -> Add/1
  Add/1 -> Product1/1
  Constant4/1 -> Product1/2
  Product1/1 -> Pressure/1, Display/1
  y/1 -> Display1/1, Subtract/1

== system pid_10/Sensor & Motor/Motor Ctrl/Subsystem ==
  note: Motor Power
  note: Motor Disable
  note: Motor Break
  note: SCL_2 = D6
      | SDA_2 = PB_11
      | U3: I2C to Analog
      | Address: 0X2A
  note: PID handles motor value
      | Not manual function
  pwr : Inport
  user : Inport  Port=2
  Data Type Conversion1 : DataTypeConversion  OutDataTypeStr=uint8  SaturateOnIntegerOverflow=off  RndMeth=Floor
  MATLAB Function : MATLAB Function  Commented=on  TreatAsAtomicUnit=on
  MATLAB Function1 : MATLAB Function  TreatAsAtomicUnit=on
  Motor Break : mbedblockslib/Digital Write  Pin=PB_0  Direction=output
      settings: SourceProductBaseCode=MICROBIT,NUCLEO,STMICRODIS
  Motor Disable : mbedblockslib/Digital Write  Pin=PB_0  Direction=output
      settings: SourceProductBaseCode=MICROBIT,NUCLEO,STMICRODIS
  Motor Power : mbedblockslib/Digital Write  Pin=PB_0  Direction=output
      settings: SourceProductBaseCode=MICROBIT,NUCLEO,STMICRODIS
  Motor Speed Control : mbedblockslib/I2C Master Write  I2CModule=2  Mode=Master  SlaveAddress=uint8(hex2dec('2A'))  SlaveByteOrder=BigEndian  Direction=Transmitter  RegisterAddressMode=on  RegisterAddress=uint8(hex2dec('10'))  SlaveDataType=uint8  DataLength=2  NoAck=off  RepeatedStart=off  OutputStatus=off
      settings: SourceProductBaseCode=MICROBIT,NUCLEO,STMICRODIS
  wires:
  MATLAB Function1/3(mtr_dis) -> Motor Disable/1
  Data Type Conversion1/1 -> Motor Speed Control/1
  pwr/1 -> MATLAB Function1/1(pwr)
  MATLAB Function1/2(mtr_brk) -> Motor Break/1
  MATLAB Function1/1(mtr_pwr) -> Motor Power/1
  user/1 -> Data Type Conversion1/1

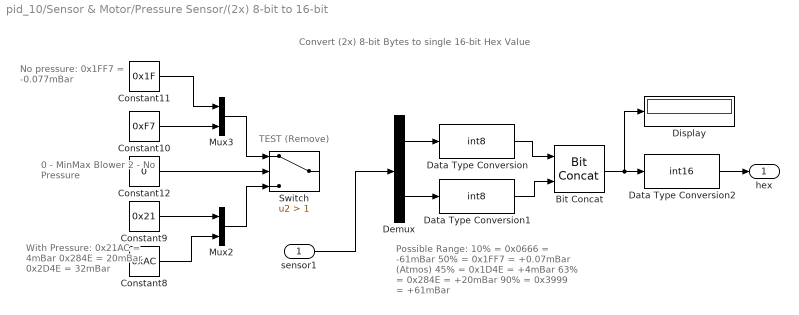
== system pid_10/Sensor & Motor/Pressure Sensor/(2x) 8-bit to 16-bit ==
  note: TEST (Remove)
  note: With Pressure:
      | 0x21AC = 4mBar
      | 0x284E = 20mBar
      | 0x2D4E = 32mBar
  note: Possible Range:
      | 10% = 0x0666 = -61mBar
      | 50% = 0x1FF7 = +0.07mBar (Atmos)
      | 45% = 0x1D4E = +4mBar
      | 63% = 0x284E = +20mBar
      | 90% = 0x3999 = +61mBar
  note: No pressure:
      | 0x1FF7 = -0.077mBar
  note: 0 - MinMax Blower
      | 2 - No Pressure
  note: Convert (2x) 8-bit Bytes to single 16-bit Hex Value
  sensor1 : Inport
  Bit Concat : hdlsllib/Logic and Bit Operations/Bit Concat  numInputs=2
  Constant10 : Constant  Value=0xF7
  Constant11 : Constant  Value=0x1F
  Constant12 : Constant  Value=0
  Constant8 : Constant  Value=0xAC
  Constant9 : Constant  Value=0x21
  Data Type Conversion : DataTypeConversion  OutDataTypeStr=int8  SaturateOnIntegerOverflow=off  RndMeth=Floor
  Data Type Conversion1 : DataTypeConversion  OutDataTypeStr=int8  SaturateOnIntegerOverflow=off  RndMeth=Floor
  Data Type Conversion2 : DataTypeConversion  OutDataTypeStr=int16  SaturateOnIntegerOverflow=off  RndMeth=Floor
  Demux : Demux  Outputs=2
  Display : Display
      settings: Format=hex (Stored Integer)
  Mux2 : Mux  Inputs=2
  Mux3 : Mux  Inputs=2
  Switch : Switch  Criteria=u2 > Threshold  Threshold=1  SaturateOnIntegerOverflow=off  InputSameDT=off
  hex : Outport
  wires:
  sensor1/1 -> Demux/1
  Data Type Conversion2/1 -> hex/1
  Mux2/1 -> Switch/3
  Mux3/1 -> Switch/1
  Constant12/1 -> Switch/2
  Constant11/1 -> Mux3/1
  Constant10/1 -> Mux3/2
  Constant8/1 -> Mux2/2
  Constant9/1 -> Mux2/1
  Bit Concat/1 -> Data Type Conversion2/1, Display/1
  Demux/2 -> Data Type Conversion1/1
  Demux/1 -> Data Type Conversion/1
  Data Type Conversion1/1 -> Bit Concat/2
  Data Type Conversion/1 -> Bit Concat/1

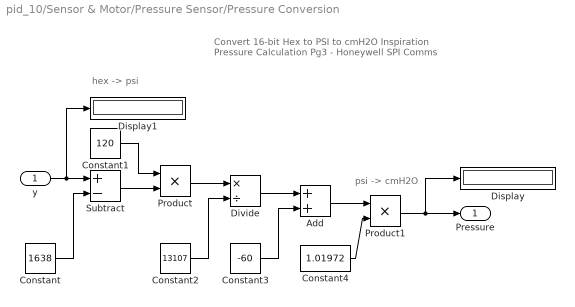
== system pid_10/Sensor & Motor/Pressure Sensor/Pressure Conversion ==
  note: hex -> psi
  note: Convert 16-bit Hex to PSI to cmH2O
      | Inspiration Pressure Calculation
      | Pg3 - Honeywell SPI Comms
  note: psi -> cmH2O
  y : Inport
  Add : Sum
  Constant : Constant  Value=1638
  Constant1 : Constant  Value=120
  Constant2 : Constant  Value=13107
  Constant3 : Constant  Value=-60
  Constant4 : Constant  Value=1.01972
  Display : Display
  Display1 : Display
      settings: Format=hex (Stored Integer)
  Divide : Product  Inputs=*/
  Product : Product
  Product1 : Product
  Subtract : Sum  Inputs=+-
  Pressure : Outport
  wires:
  y/1 -> Subtract/1, Display1/1
  Product1/1 -> Display/1, Pressure/1
  Constant4/1 -> Product1/2
  Add/1 -> Product1/1
  Divide/1 -> Add/1
  Constant3/1 -> Add/2
  Constant2/1 -> Divide/2
  Product/1 -> Divide/1
  Constant1/1 -> Product/1
  Subtract/1 -> Product/2
  Constant/1 -> Subtract/2

== matlab function pid_10/PID Tuning (ERROR)/Motor Ctrl/Subsystem/MATLAB Function ==
  data: pwr input; mtr_ctrl output; user input; mtr_pwr output; mtr_brk output; press input; mtr_dis output
function [mtr_ctrl, mtr_pwr, mtr_brk, mtr_dis] = fcn(pwr, user, press)

if pwr >= 1
    mtr_pwr = 1;
    % delay()
    mtr_brk = 1;
    mtr_dis = 1;
else
    mtr_pwr = 0;
    % delay()
    mtr_brk = 0;
    mtr_dis = 0;
end

while user >= press
    speed += 1;         % needs initial value?
    mtr_ctrl = speed;   % update speed control I2C
end

== matlab function pid_10/Working Mtr Ctrl/Motor Ctrl/MATLAB Function ==
  data: pwr input; mtr_ctrl output; user input; mtr_pwr output; mtr_brk output; press input; mtr_dis output
function [mtr_ctrl, mtr_pwr, mtr_brk, mtr_dis] = fcn(pwr, user, press)

if pwr >= 1
    mtr_pwr = 1;
    % delay()
    mtr_brk = 1;
    mtr_dis = 1;
else
    mtr_pwr = 0;
    % delay()
    mtr_brk = 0;
    mtr_dis = 0;
end

while user >= press
    speed += 1;         % needs initial value?
    mtr_ctrl = speed;   % update speed control I2C
end

== matlab function pid_10/Working Mtr Ctrl/Motor Ctrl/MATLAB Function1 ==
  data: pwr input; mtr_pwr output; mtr_brk output; mtr_dis output
function [mtr_pwr, mtr_brk, mtr_dis] = fcn(pwr)

delay = 100;

% Enable all Motor Pins
if pwr >= 1
    mtr_pwr = 1;
    % delay()
    mtr_brk = 1;
    mtr_dis = 1;
% Disable all Motor Pins
else
    mtr_dis = 0;
    mtr_brk = 0;
    pause(delay);
    mtr_pwr = 0;
end

== stateflow chart pid_10/PID Tuning (ERROR)/Motor Ctrl/LED ==
  note: TEST:
      | Routine Checks
  state Run % Parent
    state Check % Check Sub-Systems
      entry:
      LED = 0; % LED Off
      exit:
    state LED % Child
      entry: % none
      LED = 1; % LED On
      exit: % none
    (default) -> LED % Child
    LED % Child -> Check % Check Sub-Systems : after(1,sec)
    Check % Check Sub-Systems -> LED % Child : after(3,sec)
  note: Check Input
      | Power present?
  (default) -> Run % Parent
  data: LED output

== stateflow chart pid_10/Board Check/Start-Up ==
  note: TEST:
      | Routine Checks
  state Run % Parent
    state LED % Child
      entry: % none
      LED = 1; % LED On
      exit: % none
    (default) -> LED % Child
  state Check % Check Sub-Systems
    entry:
    LED = 0; % LED Off
    exit:
  note: Check Input
      | Power present?
  (default) -> Run % Parent
  Check % Check Sub-Systems -> Run % Parent : after(2,sec)
  Run % Parent -> Check % Check Sub-Systems : after(2,sec)
  data: LED output

== stateflow chart pid_10/Sensor & Motor/Motor Ctrl/LED ==
  note: TEST:
      | Routine Checks
  state Run % Parent
    state Check % Check Sub-Systems
      entry:
      LED = 0; % LED Off
      exit:
    state LED % Child
      entry: % none
      LED = 1; % LED On
      exit: % none
    (default) -> LED % Child
    LED % Child -> Check % Check Sub-Systems : after(1,sec)
    Check % Check Sub-Systems -> LED % Child : after(3,sec)
  note: Check Input
      | Power present?
  (default) -> Run % Parent
  data: LED output

== stateflow chart pid_10/Working Mtr Ctrl/Motor Ctrl/Motor_Ctrl ==
  state SHUTDOWN % Blower Off
    state Stop_1 % I2C to Anal.
      entry: mtr = 0;
      exit:
    state Stop_2 % Motor Brake
      entry:
      mtr_brk = 0; % Enable
      exit:
    state Stop_3 % Motor Disable
      entry:
      mtr_dis = 0; % Disable
      exit:
    state Stop_4 % Main Power
      entry:
      mtr_pwr = 0; % OFF
      exit:
    (default) -> Stop_1 % I2C to Anal.
    Stop_1 % I2C to Anal. -> Stop_2 % Motor Brake : after(1,sec)
    Stop_2 % Motor Brake -> Stop_3 % Motor Disable : after(500,msec)
    Stop_3 % Motor Disable -> Stop_4 % Main Power : after(1,sec)
  state STARTUP % Blower Start
    state Start_1 % Main Power
      entry:
      mtr_pwr = 0; % ON
      mtr_brk = 0; % Enabled
      mtr_dis = 0; % Disabled
      exit:
    (default) -> STARTUP.Start_1 % Main Power
  state Start_Mtr % Blower On
    state Start_1 % Main Power
      entry:
      mtr_pwr = 1; % ON
      exit:
    state Start_2 % Motor Brake
      entry:
      mtr_brk = 1; % Disable
      mtr_dis = 1; % Enabled
      exit:
    (default) -> Start_Mtr.Start_1 % Main Power
    Start_Mtr.Start_1 % Main Power -> Start_2 % Motor Brake : after(1,sec)
  state Run_Mtr % Continuous
    entry: mtr =1; % I2C output
    exit:
    note: Continuously Run the
        | Motor until Stop bit set
  note: Stop Motor after 3min
  note: Wait for Start
  note: POWER PIN:
      | Disable = <0.8V or Gnd
      | Enable = >30V or Not wired
  note: BRAKE PIN:
      | Enabled = <0.8V or Gnd
      | Deactivated = >2.4V or Not wired
  note: DISABLE PIN:
      | Disable = <0.8V or Gnd
      | Enable = >2.4V or Not wired
  note: 1. Power - On
      | 2. Brake - Off
      | 3. Disable - Off
      | 4. Voltage Output
  (default) -> STARTUP % Blower Start
  Run_Mtr % Continuous -> SHUTDOWN % Blower Off : after(5,sec)
  STARTUP % Blower Start -> (junction 53) : after(100,msec)
  (junction 53) -> Start_Mtr % Blower On [order 1] : [power == 1]
  (junction 53) -> STARTUP % Blower Start [order 2] : [power == 0]
  Start_Mtr % Blower On -> Run_Mtr % Continuous : after(2,sec)
  data: mtr output; mtr_brk output; mtr_pwr output; power input; mtr_dis output

== stateflow chart pid_10/Working Mtr Ctrl/Motor Ctrl/LED ==
  note: TEST:
      | Routine Checks
  state Run % Parent
    state Check % Check Sub-Systems
      entry:
      LED = 0; % LED Off
      exit:
    state LED % Child
      entry: % none
      LED = 1; % LED On
      exit: % none
    (default) -> LED % Child
    LED % Child -> Check % Check Sub-Systems : after(1,sec)
    Check % Check Sub-Systems -> LED % Child : after(3,sec)
  note: Check Input
      | Power present?
  (default) -> Run % Parent
  data: LED output

== stateflow chart pid_10/Sensor & Motor/Motor Ctrl/Motor_Ctrl ==
  state SHUTDOWN % Blower Off
    state Stop_1 % I2C to Anal.
      entry: mtr = 0;
      exit:
    state Stop_2 % Motor Brake
      entry:
      mtr_brk = 0; % Enable
      exit:
    state Stop_3 % Motor Disable
      entry:
      mtr_dis = 0; % Disable
      exit:
    state Stop_4 % Main Power
      entry:
      mtr_pwr = 0; % OFF
      exit:
    (default) -> Stop_1 % I2C to Anal.
    Stop_1 % I2C to Anal. -> Stop_2 % Motor Brake : after(1,sec)
    Stop_2 % Motor Brake -> Stop_3 % Motor Disable : after(500,msec)
    Stop_3 % Motor Disable -> Stop_4 % Main Power : after(1,sec)
  state STARTUP % Blower Start
    state Start_1 % Main Power
      entry:
      mtr_pwr = 0; % ON
      mtr_brk = 0; % Enabled
      mtr_dis = 0; % Disabled
      exit:
    (default) -> STARTUP.Start_1 % Main Power
  state Start_Mtr % Blower On
    state Start_1 % Main Power
      entry:
      mtr_pwr = 1; % ON
      exit:
    state Start_2 % Motor Brake
      entry:
      mtr_brk = 1; % Disable
      mtr_dis = 1; % Enabled
      exit:
    (default) -> Start_Mtr.Start_1 % Main Power
    Start_Mtr.Start_1 % Main Power -> Start_2 % Motor Brake : after(1,sec)
  state Run_Mtr % Continuous
    entry: mtr =1; % I2C output
    exit:
    note: Continuously Run the
        | Motor until Stop bit set
  note: Stop Motor after 3min
  note: Wait for Start
  note: POWER PIN:
      | Disable = <0.8V or Gnd
      | Enable = >30V or Not wired
  note: BRAKE PIN:
      | Enabled = <0.8V or Gnd
      | Deactivated = >2.4V or Not wired
  note: DISABLE PIN:
      | Disable = <0.8V or Gnd
      | Enable = >2.4V or Not wired
  note: 1. Power - On
      | 2. Brake - Off
      | 3. Disable - Off
      | 4. Voltage Output
  (default) -> STARTUP % Blower Start
  Run_Mtr % Continuous -> SHUTDOWN % Blower Off : after(5,sec)
  STARTUP % Blower Start -> (junction 53) : after(100,msec)
  (junction 53) -> Start_Mtr % Blower On [order 1] : [power == 1]
  (junction 53) -> STARTUP % Blower Start [order 2] : [power == 0]
  Start_Mtr % Blower On -> Run_Mtr % Continuous : after(2,sec)
  data: mtr output; mtr_brk output; mtr_pwr output; power input; mtr_dis output
